simulink model "CSTHMaster"  (Simulink 5.0)
settings: Solver=ode45  StartTime=0.0  StopTime=1000  MaxStep=1  RelTol=1e-3  AbsTol=1e-6
libraries: simulink_extras x3, simulink x2
settings Model: LastModifiedBy=nina  ExtModeTrigMode=oneshot  ExtModeArmWhenConnect=off  LimitDataPoints=off  BooleanDataType=off

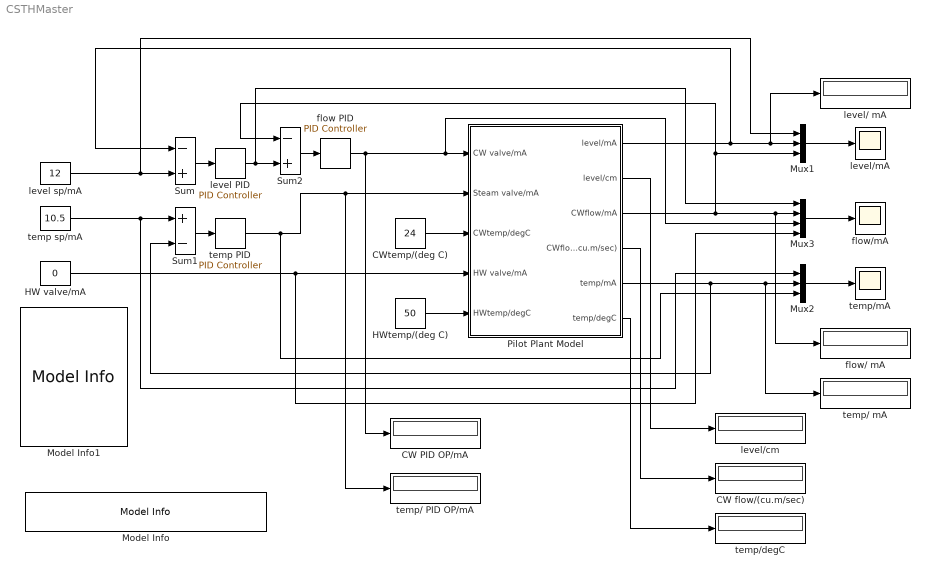
== system CSTHMaster ==
  CW PID OP/mA : Display
      settings: Format=short_e
  CW flow/(cu.m/sec) : Display
      settings: Format=short_e
  CWtemp/(deg C) : Constant  Value=24
  HW valve/mA : Constant  Value=0
  HWtemp/(deg C) : Constant  Value=50
  Model Info : simulink/Model-Wide Utilities/Model Info  InitialBlockCM=none  BlockCM=none  Frame=off  DisplayStringWithTags=Nina Thornhill, University College London September 1999, Revised November 2006  HorizontalTextAlignment=Left  LeftAlignmentValue=0.02  SourceBlockDiagram=CSTHMaster  TagMaxNumber=20
  Model Info1 : simulink/Model-Wide Utilities/Model Info  InitialBlockCM=none  BlockCM=none  Frame=off  DisplayStringWithTags=|  HorizontalTextAlignment=Left  LeftAlignmentValue=0.02  SourceBlockDiagram=CSTHMaster  TagMaxNumber=20
      | Standard operating
      | condition 1 is
      | Level sp = 12 mA
      | Temp sp = 10.5 mA
      | HW valve = 0 mA
      | 
      | Standard operating
      | condition 2 is
      | Level sp = 12 mA
      | Temp sp = 10.5 mA
      | HW valve = 5.5 mA
  Mux1 : Mux  Inputs=3
  Mux2 : Mux  Inputs=3
  Mux3 : Mux
  Pilot Plant Model : Subsystem
  Sum : Sum  Inputs=-+  SaturateOnIntegerOverflow=on  InputSameDT=on
  Sum1 : Sum  Inputs=+-  SaturateOnIntegerOverflow=on  InputSameDT=on
  Sum2 : Sum  Inputs=-+  SaturateOnIntegerOverflow=on  InputSameDT=on
  flow PID : simulink_extras/Additional Linear/PID Controller  P=0.5  I=0.2  D=0
  flow/ mA : Display
      settings: Format=short_e
  flow/mA : Scope
      settings: TimeRange=1000  YMin=2.5  YMax=25  SaveName=flow  DataFormat=Array
  level PID : simulink_extras/Additional Linear/PID Controller  P=2  I=0.1  D=0
  level sp/mA : Constant  Value=12
  level/ mA : Display
      settings: Format=short_e
  level/cm : Display
      settings: Format=short_e
  level/mA : Scope
      settings: TimeRange=1000  YMin=2.5  YMax=25  SaveName=level  DataFormat=Array
  temp PID : simulink_extras/Additional Linear/PID Controller  P=3  I=0.1  D=0
  temp sp/mA : Constant  Value=10.5
  temp/ PID OP/mA : Display
      settings: Format=short_e
  temp/ mA : Display
      settings: Format=short_e
  temp/degC : Display
      settings: Format=short_e
  temp/mA : Scope
      settings: TimeRange=1000  YMin=-35  YMax=25  SaveName=temperature  DataFormat=Array
  wires:
  Mux1/1 -> level/mA/1
  Pilot Plant Model/1(level/mA) -> Sum/1, Mux1/2, level/ mA/1
  CWtemp/(deg C)/1 -> Pilot Plant Model/3(CWtemp/degC)
  Sum/1 -> level PID/1
  level sp/mA/1 -> Sum/2, Mux1/1
  Sum1/1 -> temp PID/1
  Pilot Plant Model/5(temp/mA) -> Sum1/2, Mux2/2, temp/ mA/1
  Mux2/1 -> temp/mA/1
  temp PID/1 -> Mux2/3, Pilot Plant Model/2(Steam valve/mA), temp/ PID OP/mA/1
  Sum2/1 -> flow PID/1
  temp sp/mA/1 -> Sum1/1, Mux2/1
  Mux3/1 -> flow/mA/1
  Pilot Plant Model/3(CWflow/mA) -> Mux1/3, Sum2/1, Mux3/2, flow/ mA/1
  level PID/1 -> Sum2/2, Mux3/1
  flow PID/1 -> Pilot Plant Model/1(CW valve/mA), Mux3/3, CW PID OP/mA/1
  HWtemp/(deg C)/1 -> Pilot Plant Model/5(HWtemp/degC)
  HW valve/mA/1 -> Pilot Plant Model/4(HW valve/mA), Mux3/4
  Pilot Plant Model/2(level/cm) -> level/cm/1
  Pilot Plant Model/4(CWflow/ (cu.m/sec)) -> CW flow/(cu.m/sec)/1
  Pilot Plant Model/6(temp/degC) -> temp/degC/1

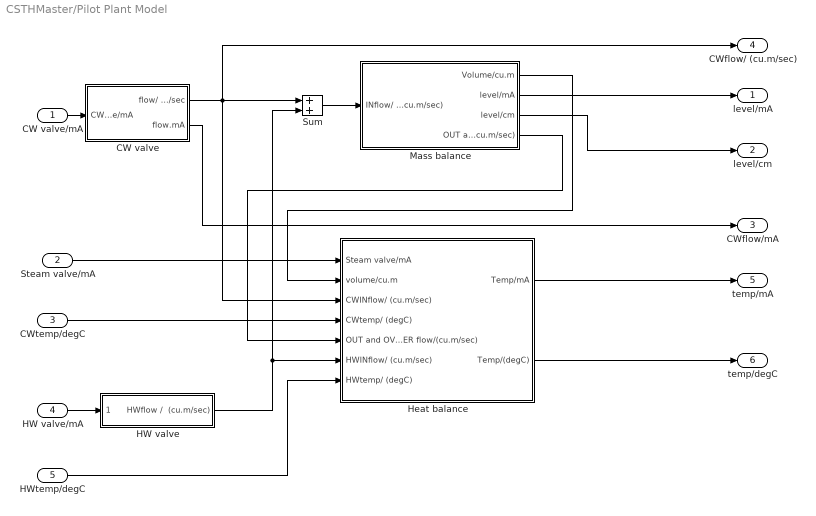
== system CSTHMaster/Pilot Plant Model ==
  CW valve/mA : Inport
  Steam valve/mA : Inport  Port=2
  CWtemp/degC : Inport  Port=3
  HW valve/mA : Inport  Port=4
  HWtemp/degC : Inport  Port=5
  CW valve : Subsystem
  HW valve : Subsystem
  Heat balance : Subsystem
  Mass balance : Subsystem
  Sum : Sum  SaturateOnIntegerOverflow=on  InputSameDT=on
  level/mA : Outport
  level/cm : Outport  Port=2
  CWflow/mA : Outport  Port=3
  CWflow/ (cu.m/sec) : Outport  Port=4
  temp/mA : Outport  Port=5
  temp/degC : Outport  Port=6
  wires:
  Mass balance/1(Volume/cu.m) -> Heat balance/2(volume/cu.m)
  CW valve/mA/1 -> CW valve/1(CWValve/mA)
  CW valve/2(flow.mA) -> CWflow/mA/1
  Steam valve/mA/1 -> Heat balance/1(Steam valve/mA)
  Heat balance/1(Temp/mA) -> temp/mA/1
  CWtemp/degC/1 -> Heat balance/4(CWtemp/ (degC))
  Heat balance/2(Temp/(degC)) -> temp/degC/1
  Mass balance/4(OUT and OVER flow/(cu.m/sec)) -> Heat balance/5(OUT and OVER flow/(cu.m/sec))
  Mass balance/2(level/mA) -> level/mA/1
  Mass balance/3(level/cm) -> level/cm/1
  HW valve/mA/1 -> HW valve/1(" ")
  CW valve/1(flow/ cu.m/sec) -> CWflow/ (cu.m/sec)/1, Sum/1, Heat balance/3(CWINflow/ (cu.m/sec))
  Sum/1 -> Mass balance/1(INflow/ (cu.m/sec))
  HW valve/1("HWflow /  (cu.m/sec) ") -> Sum/2, Heat balance/6(HWINflow/ (cu.m/sec))
  HWtemp/degC/1 -> Heat balance/7(HWtemp/ (degC))

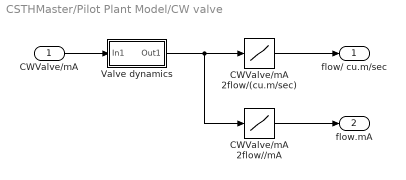
== system CSTHMaster/Pilot Plant Model/CW valve ==
  CWValve/mA : Inport
  CWValve/mA 2flow/(cu.m/sec) : Lookup  InputValues="[ 0  4  5     6     8    10    12    14    16    18    20   24]"  OutputValues="[ 0  0  1.9000e-005  2.8000e-005  4.0000e-005  5.6000e-005  7.7000e-005  1.0500e-004 1.3800e-004  1.7500e-004  2.0800e-004   2.0800e-004]"  SaturateOnIntegerOverflow=on
  CWValve/mA 2flow//mA : Lookup  InputValues="[0     3     4     5     6     7     8     9    10    11    13    15  18    21    24]"  OutputValues="[ 4.3400    4.3350    4.3350    5.7100    6.3200    6.9250    7.5000 8.0750    8.8700    9.7800   11.9400   14.6800   19.5300   24.2000  24.2000]"  SaturateOnIntegerOverflow=on
  Valve dynamics : Subsystem
  flow/ cu.m/sec : Outport
  flow.mA : Outport  Port=2
  wires:
  Valve dynamics/1(Out1) -> CWValve/mA 2flow//mA/1, CWValve/mA 2flow/(cu.m/sec)/1
  CWValve/mA/1 -> Valve dynamics/1(In1)
  CWValve/mA 2flow/(cu.m/sec)/1 -> flow/ cu.m/sec/1
  CWValve/mA 2flow//mA/1 -> flow.mA/1

== system CSTHMaster/Pilot Plant Model/HW valve ==
  " " : Inport
  HWValve/mA 2flow/(cu.m/sec) : Lookup  InputValues="[ 0    4    5     6     7      8    9      10    12 ]"  OutputValues="[ 0   0  3.07e-005  7.36e-005  11.29e-005  14.88e-005   17.87e-005   20.56e-005  23.91e-005]"  SaturateOnIntegerOverflow=on
  limit to 0 to 25 mA : Saturate  UpperLimit=25  LowerLimit=0
  "HWflow /  (cu.m/sec) " : Outport
  wires:
  HWValve/mA 2flow/(cu.m/sec)/1 -> "HWflow /  (cu.m/sec) "/1
  " "/1 -> limit to 0 to 25 mA/1
  limit to 0 to 25 mA/1 -> HWValve/mA 2flow/(cu.m/sec)/1

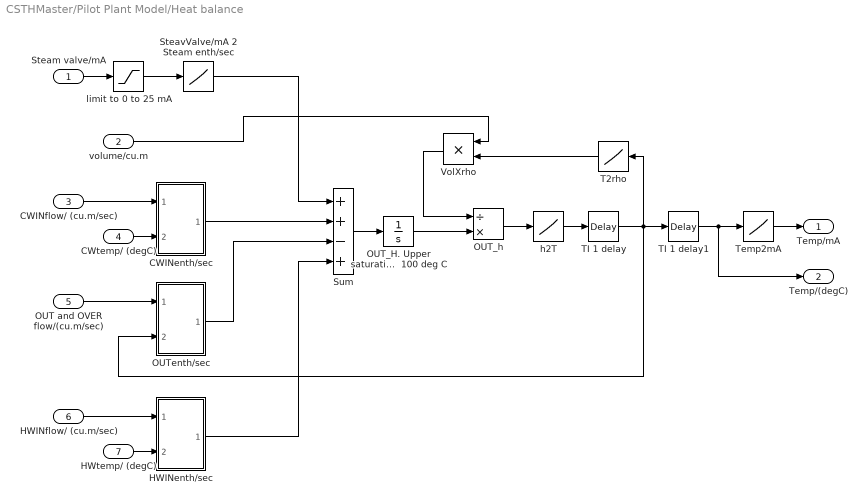
== system CSTHMaster/Pilot Plant Model/Heat balance ==
  Steam valve/mA : Inport
  volume/cu.m : Inport  Port=2
  CWINflow/ (cu.m/sec) : Inport  Port=3
  CWtemp/ (degC) : Inport  Port=4
  OUT and OVER flow/(cu.m/sec) : Inport  Port=5
  HWINflow/ (cu.m/sec) : Inport  Port=6
  HWtemp/ (degC) : Inport  Port=7
  CWINenth/sec : Subsystem
  HWINenth/sec : Subsystem
  OUT_H. Upper saturation limit is for full tank at  100 deg C : Integrator  InitialCondition=583.3  LimitOutput=on  UpperSaturationLimit=3000  LowerSaturationLimit=0
  OUT_h : Product  Inputs=/*  SaturateOnIntegerOverflow=on  InputSameDT=on
  OUTenth/sec : Subsystem
  SteavValve/mA 2 Steam enth/sec : Lookup  InputValues="[  0 ;   4.0000;    7.5000 ;   9.0000 ;  11.0000 ;  14.0000 ;  17.0000;  20.0000;  25.0000]"  OutputValues="[0 ;   0 ;   2.24;   2.61 ;   4.65 ;   8.89 ;  13.60;  15.04;  15.04]"  SaturateOnIntegerOverflow=on
  Sum : Sum  Inputs=++-+  SaturateOnIntegerOverflow=on  InputSameDT=on
  T2rho : Lookup  Orientation=left  InputValues=[0; 25; 50; 75; 100]  OutputValues=[1000; 997; 988; 975; 958]  SaturateOnIntegerOverflow=on
  TI 1 delay : TransportDelay  DelayTime=0.5
  TI 1 delay1 : TransportDelay  DelayTime=7.5
  Temp2mA : Lookup  InputValues="[24.0000   30.0000   31.0000   36.5000   44.5000   48.0000   61.0000  65.000]"  OutputValues="[7.7850    8.6100    8.7600    9.5900   10.8000   11.3800   13.52   14.2000]"  SaturateOnIntegerOverflow=on
  VolXrho : Product  Orientation=left  Inputs=**  SaturateOnIntegerOverflow=on  InputSameDT=on
  h2T : Lookup  InputValues="[25.5; 33.6; 42.0;  50.4; 62.9 ; 83.9; 104.8; 125.7; 142.4; 159.1; 175.8; 192.5; 209.3; 230.2;  251.1; 272; 293; 313.9; 334.9; 355.9; 376.9; 398; 419.1]"  OutputValues="[ 6;  8; 10; 12; 15 ;20; 25; 30; 34; 38 ; 42; 46; 50; 55; 60; 65; 70; 75; 80; 85; 90; 95; 100]"  SaturateOnIntegerOverflow=on
  limit to 0 to 25 mA : Saturate  UpperLimit=25  LowerLimit=0
  Temp/mA : Outport
  Temp/(degC) : Outport  Port=2
  wires:
  OUT_h/1 -> h2T/1
  Sum/1 -> OUT_H. Upper saturation limit is for full tank at  100 deg C/1
  SteavValve/mA 2 Steam enth/sec/1 -> Sum/1
  OUTenth/sec/1(OUT_H) -> Sum/3
  CWINenth/sec/1(IN_H) -> Sum/2
  VolXrho/1 -> OUT_h/1
  Steam valve/mA/1 -> limit to 0 to 25 mA/1
  CWINflow/ (cu.m/sec)/1 -> CWINenth/sec/1(INflow)
  CWtemp/ (degC)/1 -> CWINenth/sec/2(IN_T)
  OUT and OVER flow/(cu.m/sec)/1 -> OUTenth/sec/1(OUTflow)
  volume/cu.m/1 -> VolXrho/1
  h2T/1 -> TI 1 delay/1
  TI 1 delay/1 -> T2rho/1, OUTenth/sec/2(OUT_T), TI 1 delay1/1
  T2rho/1 -> VolXrho/2
  OUT_H. Upper saturation limit is for full tank at  100 deg C/1 -> OUT_h/2
  Temp2mA/1 -> Temp/mA/1
  TI 1 delay1/1 -> Temp2mA/1, Temp/(degC)/1
  HWINflow/ (cu.m/sec)/1 -> HWINenth/sec/1(INflow)
  HWtemp/ (degC)/1 -> HWINenth/sec/2(IN_T)
  HWINenth/sec/1(IN_H) -> Sum/4
  limit to 0 to 25 mA/1 -> SteavValve/mA 2 Steam enth/sec/1

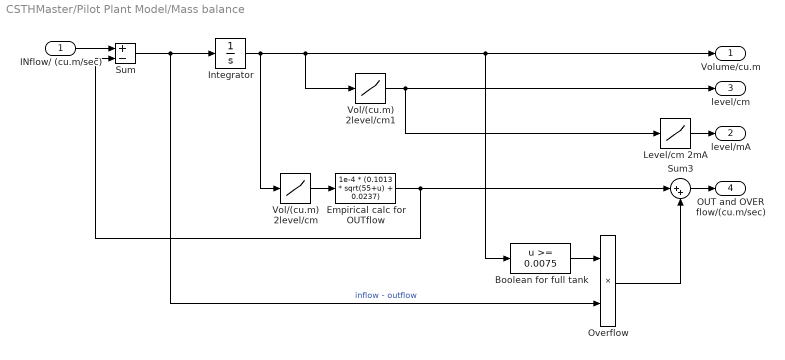
== system CSTHMaster/Pilot Plant Model/Mass balance ==
  INflow/ (cu.m/sec) : Inport
  Boolean for full tank : Fcn  Expr=u >= 0.0075
  Empirical calc for OUTflow : Fcn  Expr=1e-4 * (0.1013 * sqrt(55+u) + 0.0237)
  Integrator : Integrator  InitialCondition=0.003309  LimitOutput=on  UpperSaturationLimit=7.5*1e-3  LowerSaturationLimit=0
  Level/cm 2mA : Lookup  InputValues="[1.0000    1.6000    3.2000    4.8000    6.5000    8.3000   10.0000   11.8000   13.5000   15.3000   16.9000   18.5000   24.9000   31.2000   32.8000   34.3000   35.9000   37.5000   39.1000   40.7000   42.4000  44.0000   45.6000   47.3000]"  OutputValues="[3.5590    3.8830    4.5510    5.2930    6.0160    6.7700    7.5390  8.2850    9.0270    9.7970   10.4900   11.1700   13.8600   16.5400  17.2100   17.8800   18.5400   19.2400   19.9600   20.6300   21.3600   22.0500   22.7500   23.4700]"  SaturateOnIntegerOverflow=on
  Overflow : Product  SaturateOnIntegerOverflow=on
  Sum : Sum  Inputs=+-  SaturateOnIntegerOverflow=on  InputSameDT=on
  Sum3 : Sum  Inputs=|++  SaturateOnIntegerOverflow=on
  Vol/(cu.m) 2level/cm : Lookup  InputValues="1e-3*[0    0.2500    0.5000    0.7500    1.0000    1.2500    1.5000  1.7500    2.0000    2.5000    2.7500    3.0000    4.0000    5.0000  5.2500    5.5000    5.7500    6.0000    6.2500    6.5000    6.7500   7.0000    7.2500    7.5000]"  OutputValues="[1.0000    1.6000    3.2000    4.8000    6.5000    8.3000   10.0000   11.8000   13.5000   15.3000   16.9000   18.5000   24.9000   31.2000   32.8000   34.3000   35.9000   37.5000   39.1000   40.7000   42.4000  44.0000   45.6000   47.3000]"  SaturateOnIntegerOverflow=on
  Vol/(cu.m) 2level/cm1 : Lookup  InputValues="1e-3*[0    0.2500    0.5000    0.7500    1.0000    1.2500    1.5000  1.7500    2.0000    2.5000    2.7500    3.0000    4.0000    5.0000  5.2500    5.5000    5.7500    6.0000    6.2500    6.5000    6.7500   7.0000    7.2500    7.5000]"  OutputValues="[1.0000    1.6000    3.2000    4.8000    6.5000    8.3000   10.0000   11.8000   13.5000   15.3000   16.9000   18.5000   24.9000   31.2000   32.8000   34.3000   35.9000   37.5000   39.1000   40.7000   42.4000  44.0000   45.6000   47.3000]"  SaturateOnIntegerOverflow=on
  Volume/cu.m : Outport
  level/mA : Outport  Port=2
  level/cm : Outport  Port=3
  OUT and OVER flow/(cu.m/sec) : Outport  Port=4
  wires:
  Sum/1 -> Integrator/1, Overflow/2  "inflow - outflow"
  INflow/ (cu.m/sec)/1 -> Sum/1
  Integrator/1 -> Vol/(cu.m) 2level/cm/1, Vol/(cu.m) 2level/cm1/1, Volume/cu.m/1, Boolean for full tank/1
  Vol/(cu.m) 2level/cm/1 -> Empirical calc for OUTflow/1
  Empirical calc for OUTflow/1 -> Sum/2, Sum3/1
  Level/cm 2mA/1 -> level/mA/1
  Vol/(cu.m) 2level/cm1/1 -> level/cm/1, Level/cm 2mA/1
  Boolean for full tank/1 -> Overflow/1
  Sum3/1 -> OUT and OVER flow/(cu.m/sec)/1
  Overflow/1 -> Sum3/2

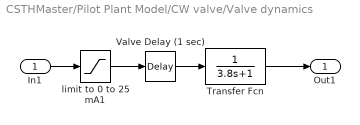
== system CSTHMaster/Pilot Plant Model/CW valve/Valve dynamics ==
  In1 : Inport
  Transfer Fcn : TransferFcn  Numerator=1  Denominator=[3.8 1]
  Valve Delay (1 sec) : TransportDelay
  limit to 0 to 25 mA1 : Saturate  UpperLimit=25  LowerLimit=0
  Out1 : Outport
  wires:
  In1/1 -> limit to 0 to 25 mA1/1
  limit to 0 to 25 mA1/1 -> Valve Delay (1 sec)/1
  Transfer Fcn/1 -> Out1/1
  Valve Delay (1 sec)/1 -> Transfer Fcn/1

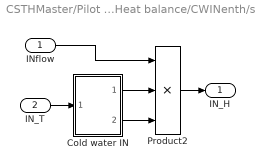
== system CSTHMaster/Pilot Plant Model/Heat balance/CWINenth/sec ==
  INflow : Inport
  IN_T : Inport  Port=2
  Cold water IN : Subsystem
  Product2 : Product  Inputs=***  SaturateOnIntegerOverflow=on  InputSameDT=on
  IN_H : Outport
  wires:
  Cold water IN/1(IN_rho) -> Product2/2
  Cold water IN/2(IN_h) -> Product2/3
  Product2/1 -> IN_H/1
  IN_T/1 -> Cold water IN/1(IN-T)
  INflow/1 -> Product2/1

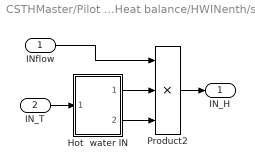
== system CSTHMaster/Pilot Plant Model/Heat balance/HWINenth/sec ==
  INflow : Inport
  IN_T : Inport  Port=2
  Hot  water IN : Subsystem
  Product2 : Product  Inputs=***  SaturateOnIntegerOverflow=on  InputSameDT=on
  IN_H : Outport
  wires:
  INflow/1 -> Product2/1
  IN_T/1 -> Hot  water IN/1(IN-T)
  Product2/1 -> IN_H/1
  Hot  water IN/2(IN_h) -> Product2/3
  Hot  water IN/1(IN_rho) -> Product2/2

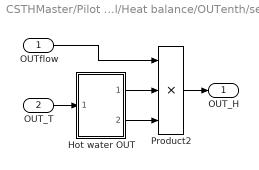
== system CSTHMaster/Pilot Plant Model/Heat balance/OUTenth/sec ==
  OUTflow : Inport
  OUT_T : Inport  Port=2
  Hot water OUT : Subsystem
  Product2 : Product  Inputs=***  SaturateOnIntegerOverflow=on  InputSameDT=on
  OUT_H : Outport
  wires:
  OUTflow/1 -> Product2/1
  OUT_T/1 -> Hot water OUT/1(OUT_T)
  Product2/1 -> OUT_H/1
  Hot water OUT/2(OUT_h) -> Product2/3
  Hot water OUT/1(OUT_rho) -> Product2/2

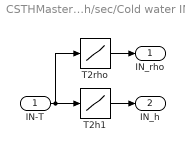
== system CSTHMaster/Pilot Plant Model/Heat balance/CWINenth/sec/Cold water IN ==
  IN-T : Inport
  T2h1 : Lookup  InputValues="[ 6;  8; 10; 12; 15 ;20; 25; 30; 34; 38 ; 42; 46; 50; 55; 60; 65; 70; 75; 80; 85; 90; 95; 100]"  OutputValues="[25.5; 33.6; 42.0;  50.4; 62.9 ; 83.9; 104.8; 125.7; 142.4; 159.1; 175.8; 192.5; 209.3; 230.2;  251.1; 272; 293; 313.9; 334.9; 355.9; 376.9; 398; 419.1]"  SaturateOnIntegerOverflow=on
  T2rho : Lookup  InputValues=[0; 25; 50; 75; 100]  OutputValues=[1000; 997; 988; 975; 958]  SaturateOnIntegerOverflow=on
  IN_rho : Outport
  IN_h : Outport  Port=2
  wires:
  IN-T/1 -> T2h1/1, T2rho/1
  T2rho/1 -> IN_rho/1
  T2h1/1 -> IN_h/1

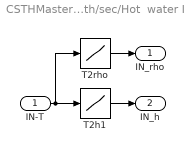
== system CSTHMaster/Pilot Plant Model/Heat balance/HWINenth/sec/Hot  water IN ==
  IN-T : Inport
  T2h1 : Lookup  InputValues="[ 6;  8; 10; 12; 15 ;20; 25; 30; 34; 38 ; 42; 46; 50; 55; 60; 65; 70; 75; 80; 85; 90; 95; 100]"  OutputValues="[25.5; 33.6; 42.0;  50.4; 62.9 ; 83.9; 104.8; 125.7; 142.4; 159.1; 175.8; 192.5; 209.3; 230.2;  251.1; 272; 293; 313.9; 334.9; 355.9; 376.9; 398; 419.1]"  SaturateOnIntegerOverflow=on
  T2rho : Lookup  InputValues=[0; 25; 50; 75; 100]  OutputValues=[1000; 997; 988; 975; 958]  SaturateOnIntegerOverflow=on
  IN_rho : Outport
  IN_h : Outport  Port=2
  wires:
  T2h1/1 -> IN_h/1
  T2rho/1 -> IN_rho/1
  IN-T/1 -> T2rho/1, T2h1/1

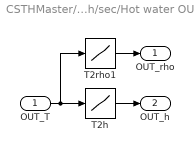
== system CSTHMaster/Pilot Plant Model/Heat balance/OUTenth/sec/Hot water OUT ==
  OUT_T : Inport
  T2h : Lookup  InputValues="[ 6;  8; 10; 12; 15 ;20; 25; 30; 34; 38 ; 42; 46; 50; 55; 60; 65; 70; 75; 80; 85; 90; 95; 100]"  OutputValues="[25.5; 33.6; 42.0;  50.4; 62.9 ; 83.9; 104.8; 125.7; 142.4; 159.1; 175.8; 192.5; 209.3; 230.2;  251.1; 272; 293; 313.9; 334.9; 355.9; 376.9; 398; 419.1]"  SaturateOnIntegerOverflow=on
  T2rho1 : Lookup  InputValues=[0; 25; 50; 75; 100]  OutputValues=[1000; 997; 988; 975; 958]  SaturateOnIntegerOverflow=on
  OUT_rho : Outport
  OUT_h : Outport  Port=2
  wires:
  OUT_T/1 -> T2h/1, T2rho1/1
  T2rho1/1 -> OUT_rho/1
  T2h/1 -> OUT_h/1
